simulink model "Two_point_distance_calculate"  (R2021a)
settings: configuration reference "AION_IDS_Speedgoat" (kept outside this file)
libraries: simulink x1
Description:
  | 计算两点之间的距离
settings Model: DataDictionary=Two_Point_Distance_Calculate.sldd  Creator=xinrui  LastModifiedBy=Administrator
settings ConfigSetRef: SourceName=AION_IDS_Speedgoat

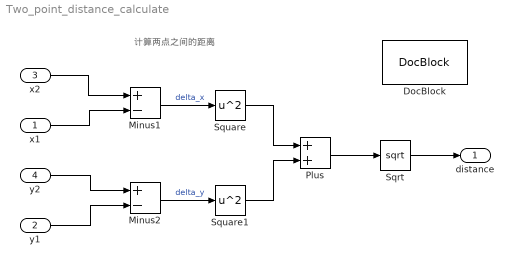
== system Two_point_distance_calculate ==
  note: 计算两点之间的距离
  x1 : Inport  Description=第一个点的x坐标，实数，m。  OutDataTypeStr=double  PortDimensions=1
  y1 : Inport  Description=第一个点的y坐标，实数，m。  Port=2  OutDataTypeStr=double  PortDimensions=1
  x2 : Inport  Description=第二个点的x坐标，实数，m。  Port=3  OutDataTypeStr=double  PortDimensions=1
  y2 : Inport  Description=第二个点的y坐标，实数，m。  Port=4  OutDataTypeStr=double  PortDimensions=1
  DocBlock : simulink/Model-Wide Utilities/DocBlock  DocumentType=HTML  mask(DocBlock){}
      mask Display:
      | plot([.8 0 0 1 1 .8 .8 1],[1 1 0 0 .8 1 .8 .8]);
      | text(.5,.6,'CHANGELOG','horizontalalignment','center');
      | text(.95,.05,get_param(gcb,'DocumentType'),'verticalalignment','bottom','horizontalalignment','right');
  Minus1 : Sum  Description=计算两点之间的x坐标增量。  Inputs=+-
  Minus2 : Sum  Description=计算两点之间的y坐标增量。  Inputs=+-
  Plus : Sum
  Sqrt : Sqrt  Description=按照公式计算两点之间的距离。  SaturateOnIntegerOverflow=on
  Square : Math  Operator=square  SaturateOnIntegerOverflow=on
  Square1 : Math  Operator=square  SaturateOnIntegerOverflow=on
  distance : Outport  Description=两点之间的距离，正实数，m。
  wires:
  x2/1 -> Minus1/1
  y2/1 -> Minus2/1
  x1/1 -> Minus1/2
  y1/1 -> Minus2/2
  Minus1/1 -> Square/1  "delta_x"
  Minus2/1 -> Square1/1  "delta_y"
  Square/1 -> Plus/1
  Square1/1 -> Plus/2
  Plus/1 -> Sqrt/1
  Sqrt/1 -> distance/1
